simulink model "My_Model"  (R2022a)
settings: Solver=VariableStepAuto  StartTime=0.0  StopTime=10.0  RelTol=1e-3
libraries: neural x1294, spsSeriesRLCBranchLib x16, spsDiodeLib x14, spsMosfetLib x9, spsVoltageMeasurementLib x9, powerlib_extras x8, spsThreePhaseVIMeasurementLib x7, spsCurrentMeasurementLib x4, spsPVArrayLib x4, spsPWMGeneratorDCDCLib x4, spsTHDLib x4, spsThreePhaseParallelRLCBranchLib x3
(part 18 of 41)

== system My_Model/Subsystem1/Custom Neural Network1/Layer 5/IW{5,1} ==
  "pd{5,1}" : Inport  PortDimensions=2
      mask Display: e = 0.06;c1 = [120 230 180]/255;c2 = ([120 230 180]+0)/(256+128);c3 = ([120 230 180]+128)/(256+128);patch([0 1 1 0],[0 0 1 1],c1);patch([0 1 1 1-e 1-e 0+e],[0 0 1 1-e 0+e 0+e],c2);patch([0 0 1 1-e 0+e 0+e],[0 1 1 1-e 1-e 0+e],c3);plot([0 1 1 0 0],[0 0 1 1 0]);
  "IW{5,1}(1,:)'" : Constant  Value=[-0.01556453275093380543558918560620440985076129436492919921875;5.4972936922844959435792422386413136337068863213062286376953125e-05]
      mask Display: e = 0.06;c1 = [120 150 230]/255;c2 = ([120 150 230]+0)/383;c3 = ([120 150 230]+128)/383;patch([0 1 1 0],[0 0 1 1],c1);patch([0 1 1 1-e 1-e 0+e],[0 0 1 1-e 0+e 0+e],c2);patch([0 0 1 1-e 0+e 0+e],[0 1 1 1-e 1-e 0+e],c3);plot([0 1 1 0 0],[0 0 1 1 0]);disp('Weights');
  "IW{5,1}(2,:)'" : Constant  Value=[-0.00943826331659743111845983776220236904919147491455078125;-0.0251008390325845910651114678557860315777361392974853515625]
      mask Display: e = 0.06;c1 = [120 150 230]/255;c2 = ([120 150 230]+0)/383;c3 = ([120 150 230]+128)/383;patch([0 1 1 0],[0 0 1 1],c1);patch([0 1 1 1-e 1-e 0+e],[0 0 1 1-e 0+e 0+e],c2);patch([0 0 1 1-e 0+e 0+e],[0 1 1 1-e 1-e 0+e],c3);plot([0 1 1 0 0],[0 0 1 1 0]);disp('Weights');
  "IW{5,1}(3,:)'" : Constant  Value=[0.001691875226755712967319222883588736294768750667572021484375;0.01000054813071515023847890546448979876004159450531005859375]
      mask Display: e = 0.06;c1 = [120 150 230]/255;c2 = ([120 150 230]+0)/383;c3 = ([120 150 230]+128)/383;patch([0 1 1 0],[0 0 1 1],c1);patch([0 1 1 1-e 1-e 0+e],[0 0 1 1-e 0+e 0+e],c2);patch([0 0 1 1-e 0+e 0+e],[0 1 1 1-e 1-e 0+e],c3);plot([0 1 1 0 0],[0 0 1 1 0]);disp('Weights');
  "IW{5,1}(4,:)'" : Constant  Value=[0.00932793326903941753813764847791389911435544490814208984375;0.01364668381544361687451871745224707410670816898345947265625]
      mask Display: e = 0.06;c1 = [120 150 230]/255;c2 = ([120 150 230]+0)/383;c3 = ([120 150 230]+128)/383;patch([0 1 1 0],[0 0 1 1],c1);patch([0 1 1 1-e 1-e 0+e],[0 0 1 1-e 0+e 0+e],c2);patch([0 0 1 1-e 0+e 0+e],[0 1 1 1-e 1-e 0+e],c3);plot([0 1 1 0 0],[0 0 1 1 0]);disp('Weights');
  "IW{5,1}(5,:)'" : Constant  Value=[-0.002392923396249546121039575297118062735535204410552978515625;-0.026184378671104908964384350156251457519829273223876953125]
      mask Display: e = 0.06;c1 = [120 150 230]/255;c2 = ([120 150 230]+0)/383;c3 = ([120 150 230]+128)/383;patch([0 1 1 0],[0 0 1 1],c1);patch([0 1 1 1-e 1-e 0+e],[0 0 1 1-e 0+e 0+e],c2);patch([0 0 1 1-e 0+e 0+e],[0 1 1 1-e 1-e 0+e],c3);plot([0 1 1 0 0],[0 0 1 1 0]);disp('Weights');
  Mux : Mux  Inputs=5
      mask Display: e = 0.06;c1 = [120 150 230]/255;c2 = ([120 150 230]+0)/383;c3 = ([120 150 230]+128)/383;patch([0 1 1 0],[0 0 1 1],c1);patch([0 1 1 1-e 1-e 0+e],[0 0 1 1-e 0+e 0+e],c2);patch([0 0 1 1-e 0+e 0+e],[0 1 1 1-e 1-e 0+e],c3);plot([0 1 1 0 0],[0 0 1 1 0]);disp('Mux');
  dotprod{1..5} (5 alike) : neural/Weight Functions/dotprod
  "iz{5,1}" : Outport
      mask Display: e = 0.06;c1 = [120 230 180]/255;c2 = ([120 230 180]+0)/(256+128);c3 = ([120 230 180]+128)/(256+128);patch([0 1 1 0],[0 0 1 1],c1);patch([0 1 1 1-e 1-e 0+e],[0 0 1 1-e 0+e 0+e],c2);patch([0 0 1 1-e 0+e 0+e],[0 1 1 1-e 1-e 0+e],c3);plot([0 1 1 0 0],[0 0 1 1 0]);
  wires:
  Mux/1 -> "iz{5,1}"/1
  dotprod5/1 -> Mux/5
  "IW{5,1}(5,:)'"/1 -> dotprod5/1
  dotprod4/1 -> Mux/4
  "IW{5,1}(4,:)'"/1 -> dotprod4/1
  dotprod3/1 -> Mux/3
  "IW{5,1}(3,:)'"/1 -> dotprod3/1
  dotprod2/1 -> Mux/2
  "IW{5,1}(2,:)'"/1 -> dotprod2/1
  dotprod1/1 -> Mux/1
  "pd{5,1}"/1 -> dotprod5/2, dotprod4/2, dotprod3/2, dotprod2/2, dotprod1/2
  "IW{5,1}(1,:)'"/1 -> dotprod1/1

== system My_Model/Subsystem1/Custom Neural Network1/Layer 5/LW{5,1} ==
  "ad{5,1}" : Inport  PortDimensions=5
      mask Display: e = 0.06;c1 = [120 230 180]/255;c2 = ([120 230 180]+0)/(256+128);c3 = ([120 230 180]+128)/(256+128);patch([0 1 1 0],[0 0 1 1],c1);patch([0 1 1 1-e 1-e 0+e],[0 0 1 1-e 0+e 0+e],c2);patch([0 0 1 1-e 0+e 0+e],[0 1 1 1-e 1-e 0+e],c3);plot([0 1 1 0 0],[0 0 1 1 0]);
  "IW{5,1}(1,:)'" : Constant  Value=[0.198320715847589756908320168804493732750415802001953125;-0.76675737162833801363603924983181059360504150390625;1.08955055179509141538574112928472459316253662109375;-0.2713503308288773840928342906408943235874176025390625;-0.6565776104818485947589579154737293720245361328125]
      mask Display: e = 0.06;c1 = [120 150 230]/255;c2 = ([120 150 230]+0)/383;c3 = ([120 150 230]+128)/383;patch([0 1 1 0],[0 0 1 1],c1);patch([0 1 1 1-e 1-e 0+e],[0 0 1 1-e 0+e 0+e],c2);patch([0 0 1 1-e 0+e 0+e],[0 1 1 1-e 1-e 0+e],c3);plot([0 1 1 0 0],[0 0 1 1 0]);disp('weights');
  "IW{5,1}(2,:)'" : Constant  Value=[0.0779959574242100328600457714856020174920558929443359375;-0.10003962086747404669484495798315037973225116729736328125;1.0731906798303751937595507115474902093410491943359375;0.000534257552850309481821955426283921042340807616710662841796875;0.413508652564843204313405067296116612851619720458984375]
      mask Display: e = 0.06;c1 = [120 150 230]/255;c2 = ([120 150 230]+0)/383;c3 = ([120 150 230]+128)/383;patch([0 1 1 0],[0 0 1 1],c1);patch([0 1 1 1-e 1-e 0+e],[0 0 1 1-e 0+e 0+e],c2);patch([0 0 1 1-e 0+e 0+e],[0 1 1 1-e 1-e 0+e],c3);plot([0 1 1 0 0],[0 0 1 1 0]);disp('weights');
  "IW{5,1}(3,:)'" : Constant  Value=[0.0464276696923932308269655777621665038168430328369140625;-0.191886394147698258194623122108168900012969970703125;-0.3521992231427344410832347421091981232166290283203125;0.64609742274914416793052396315033547580242156982421875;1.0262809271427844048929500786471180617809295654296875]
      mask Display: e = 0.06;c1 = [120 150 230]/255;c2 = ([120 150 230]+0)/383;c3 = ([120 150 230]+128)/383;patch([0 1 1 0],[0 0 1 1],c1);patch([0 1 1 1-e 1-e 0+e],[0 0 1 1-e 0+e 0+e],c2);patch([0 0 1 1-e 0+e 0+e],[0 1 1 1-e 1-e 0+e],c3);plot([0 1 1 0 0],[0 0 1 1 0]);disp('weights');
  "IW{5,1}(4,:)'" : Constant  Value=[0.98375907186508115831458098909934051334857940673828125;-0.1830940829093224142543050447784480638802051544189453125;0.9452581550422547440604148505371995270252227783203125;-0.320309813947215082929886875717784278094768524169921875;-0.73154898069945961669446887754020281136035919189453125]
      mask Display: e = 0.06;c1 = [120 150 230]/255;c2 = ([120 150 230]+0)/383;c3 = ([120 150 230]+128)/383;patch([0 1 1 0],[0 0 1 1],c1);patch([0 1 1 1-e 1-e 0+e],[0 0 1 1-e 0+e 0+e],c2);patch([0 0 1 1-e 0+e 0+e],[0 1 1 1-e 1-e 0+e],c3);plot([0 1 1 0 0],[0 0 1 1 0]);disp('weights');
  "IW{5,1}(5,:)'" : Constant  Value=[0.25564330598621010093296490595093928277492523193359375;-0.09094017318610138345125193382045836187899112701416015625;-0.436280716359431774975519147119484841823577880859375;-0.348300498410330672260926121452939696609973907470703125;0.93083543676170144021142505152965895831584930419921875]
      mask Display: e = 0.06;c1 = [120 150 230]/255;c2 = ([120 150 230]+0)/383;c3 = ([120 150 230]+128)/383;patch([0 1 1 0],[0 0 1 1],c1);patch([0 1 1 1-e 1-e 0+e],[0 0 1 1-e 0+e 0+e],c2);patch([0 0 1 1-e 0+e 0+e],[0 1 1 1-e 1-e 0+e],c3);plot([0 1 1 0 0],[0 0 1 1 0]);disp('weights');
  Mux : Mux  Inputs=5
      mask Display: e = 0.06;c1 = [120 150 230]/255;c2 = ([120 150 230]+0)/383;c3 = ([120 150 230]+128)/383;patch([0 1 1 0],[0 0 1 1],c1);patch([0 1 1 1-e 1-e 0+e],[0 0 1 1-e 0+e 0+e],c2);patch([0 0 1 1-e 0+e 0+e],[0 1 1 1-e 1-e 0+e],c3);plot([0 1 1 0 0],[0 0 1 1 0]);disp('Mux');
  dotprod{1..5} (5 alike) : neural/Weight Functions/dotprod
  "lz{5,1}" : Outport
      mask Display: e = 0.06;c1 = [120 230 180]/255;c2 = ([120 230 180]+0)/(256+128);c3 = ([120 230 180]+128)/(256+128);patch([0 1 1 0],[0 0 1 1],c1);patch([0 1 1 1-e 1-e 0+e],[0 0 1 1-e 0+e 0+e],c2);patch([0 0 1 1-e 0+e 0+e],[0 1 1 1-e 1-e 0+e],c3);plot([0 1 1 0 0],[0 0 1 1 0]);
  wires:
  Mux/1 -> "lz{5,1}"/1
  dotprod5/1 -> Mux/5
  "IW{5,1}(5,:)'"/1 -> dotprod5/1
  dotprod4/1 -> Mux/4
  "IW{5,1}(4,:)'"/1 -> dotprod4/1
  dotprod3/1 -> Mux/3
  "IW{5,1}(3,:)'"/1 -> dotprod3/1
  dotprod2/1 -> Mux/2
  "IW{5,1}(2,:)'"/1 -> dotprod2/1
  dotprod1/1 -> Mux/1
  "ad{5,1}"/1 -> dotprod5/2, dotprod4/2, dotprod3/2, dotprod2/2, dotprod1/2
  "IW{5,1}(1,:)'"/1 -> dotprod1/1

== system My_Model/Subsystem1/Custom Neural Network1/Layer 5/LW{5,2} ==
  "ad{5,2}" : Inport  PortDimensions=20
      mask Display: e = 0.06;c1 = [120 230 180]/255;c2 = ([120 230 180]+0)/(256+128);c3 = ([120 230 180]+128)/(256+128);patch([0 1 1 0],[0 0 1 1],c1);patch([0 1 1 1-e 1-e 0+e],[0 0 1 1-e 0+e 0+e],c2);patch([0 0 1 1-e 0+e 0+e],[0 1 1 1-e 1-e 0+e],c3);plot([0 1 1 0 0],[0 0 1 1 0]);
  "IW{5,2}(1,:)'" : Constant  Value=[-0.1684832167230098931565152042821864597499370574951171875;-0.158311694875728659059888059346121735870838165283203125;0.03144274628571579188740514609889942221343517303466796875;0.58926160433097063418017569347284734249114990234375;0.9422248117175568982162303655059076845645904541015625;-0.7561502004801388121535410391516052186489105224609375;0.2469253151334374896119783215908682905137538909912109375;0.36342459520089909208451217637048102915287017822265625;0.34969813386813874966918547215755097568035125732421875;-0.75124035402883071466106912339455448091030120849609375;-1.200718051335563085757485168869607150554656982421875;1.0762949692530996426143019562005065381526947021484375;1.1023353041015584441453256658860482275485992431640625;-0.267493816107898629841344018132076598703861236572265625;-0.81521522741978114101613073216867633163928985595703125;-1.037383369655141773790774095687083899974822998046875;0.27978157127544756033188377841725014150142669677734375;1.1838317043498267633339082749444060027599334716796875;-0.2358763441495083379439989812453859485685825347900390625;0.1897216833489547838098587817512452602386474609375]
      mask Display: e = 0.06;c1 = [120 150 230]/255;c2 = ([120 150 230]+0)/383;c3 = ([120 150 230]+128)/383;patch([0 1 1 0],[0 0 1 1],c1);patch([0 1 1 1-e 1-e 0+e],[0 0 1 1-e 0+e 0+e],c2);patch([0 0 1 1-e 0+e 0+e],[0 1 1 1-e 1-e 0+e],c3);plot([0 1 1 0 0],[0 0 1 1 0]);disp('weights');
  "IW{5,2}(2,:)'" : Constant  Value=[0.5812767377017793446469795526354573667049407958984375;-0.58065264983084985406236455673933960497379302978515625;-0.53889712674579726137125135210226289927959442138671875;0.455212321068005021373892304836772382259368896484375;0.381546915238895001376562277073389850556850433349609375;-0.9898117600722893261178114698850549757480621337890625;-0.036772065646242212133554261299650534056127071380615234375;0.344368316606951607727893360788584686815738677978515625;0.37959793987010959082084582405514083802700042724609375;0.99126589260002884174127757432870566844940185546875;-0.99833075074241206525726965992362238466739654541015625;0.934549989284991777793720757472328841686248779296875;-0.042023664020545518915650262670169468037784099578857421875;-0.50812566427233230026416777036502026021480560302734375;0.8581247546815966575906031721387989819049835205078125;-1.1160299752370683723512456708704121410846710205078125;-0.26941229108102737743735133335576392710208892822265625;-0.45029337265439028925584352691657841205596923828125;-0.12270439641062207136723571920811082236468791961669921875;0.492220096251096694839333167692529968917369842529296875]
      mask Display: e = 0.06;c1 = [120 150 230]/255;c2 = ([120 150 230]+0)/383;c3 = ([120 150 230]+128)/383;patch([0 1 1 0],[0 0 1 1],c1);patch([0 1 1 1-e 1-e 0+e],[0 0 1 1-e 0+e 0+e],c2);patch([0 0 1 1-e 0+e 0+e],[0 1 1 1-e 1-e 0+e],c3);plot([0 1 1 0 0],[0 0 1 1 0]);disp('weights');
  "IW{5,2}(3,:)'" : Constant  Value=[-0.1648517007952392809944086593532119877636432647705078125;-0.35915922041747305737402484737685881555080413818359375;-1.1402981796676645576127384629216976463794708251953125;-0.27685202188738078366014860876020975410938262939453125;0.392134378238151837248182118855766020715236663818359375;1.217305601499260259146240059635601937770843505859375;0.4563227505947524687002214704989455640316009521484375;-0.60795376192282446492498593215714208781719207763671875;-1.2351866808087625937417897148407064378261566162109375;-0.304290353056002105258670553666888736188411712646484375;-0.0281049809085356337712280350160654052160680294036865234375;-0.07228816906939468378556767902409774251282215118408203125;-0.0274877397507839980883570518699343665502965450286865234375;0.2313225831755712780246625470681465230882167816162109375;-0.44365232337631421710710810657474212348461151123046875;-0.5191098010197474632576586373033933341503143310546875;0.310823132335534768611040590258198790252208709716796875;0.7164023227649478631207102807820774614810943603515625;0.6809741715773840464720478848903439939022064208984375;-0.8507340797159843592822880964376963675022125244140625]
      mask Display: e = 0.06;c1 = [120 150 230]/255;c2 = ([120 150 230]+0)/383;c3 = ([120 150 230]+128)/383;patch([0 1 1 0],[0 0 1 1],c1);patch([0 1 1 1-e 1-e 0+e],[0 0 1 1-e 0+e 0+e],c2);patch([0 0 1 1-e 0+e 0+e],[0 1 1 1-e 1-e 0+e],c3);plot([0 1 1 0 0],[0 0 1 1 0]);disp('weights');
  "IW{5,2}(4,:)'" : Constant  Value=[0.6350658920207326030293870644527487456798553466796875;0.78502750463090731347648443261277861893177032470703125;0.762793473272745270463701672269962728023529052734375;0.37784362235353541326077220219303853809833526611328125;-0.192588124811389704849062809444149024784564971923828125;0.77541139946467751986602934266556985676288604736328125;0.61832300773275472582923839581781066954135894775390625;-0.7310412564267725343825077288784086704254150390625;-0.5449629474225596847958286161883734166622161865234375;1.1444776365309892174337846881826408207416534423828125;-0.050150885878106822579614032520112232305109500885009765625;0.6877296369174070722607439165585674345493316650390625;-0.39848068932220515048214792841463349759578704833984375;0.236964859673772565429317182861268520355224609375;0.1226832073435409620199010305441333912312984466552734375;-0.76214660363326203196265851147472858428955078125;-0.98776348259720714306553190908743999898433685302734375;1.055032779571795753525975669617764651775360107421875;-1.09102444565933875963992250035516917705535888671875;0.79757981845308645318937124102376401424407958984375]
      mask Display: e = 0.06;c1 = [120 150 230]/255;c2 = ([120 150 230]+0)/383;c3 = ([120 150 230]+128)/383;patch([0 1 1 0],[0 0 1 1],c1);patch([0 1 1 1-e 1-e 0+e],[0 0 1 1-e 0+e 0+e],c2);patch([0 0 1 1-e 0+e 0+e],[0 1 1 1-e 1-e 0+e],c3);plot([0 1 1 0 0],[0 0 1 1 0]);disp('weights');
  "IW{5,2}(5,:)'" : Constant  Value=[-0.529727220867986403618488111533224582672119140625;0.70651597831416446116037377578322775661945343017578125;-1.047591944087713500266545452177524566650390625;-0.405419647769215740762405175701132975518703460693359375;-1.0223374069193038593539313296787440776824951171875;-0.66965658547109130349639372070669196546077728271484375;-0.291852462499349540880899667172343470156192779541015625;0.65359162375761403751539546647109091281890869140625;-0.16324908144528327280653456909931264817714691162109375;-0.6050588281762083742165714284055866301059722900390625;-0.1199441337484412339886574727643164806067943572998046875;-0.532459193107392980692793571506626904010772705078125;0.5539672672926834184892186385695822536945343017578125;-0.65825035682826638083753323371638543903827667236328125;-0.469079745718143925614640465937554836273193359375;-0.961416751874887065554275977774523198604583740234375;-1.0711718673191363837560174943064339458942413330078125;0.65147983239813544997787175816483795642852783203125;-0.033235468255095899914319801382589503191411495208740234375;-0.69039012441932900987495713707176037132740020751953125]
      mask Display: e = 0.06;c1 = [120 150 230]/255;c2 = ([120 150 230]+0)/383;c3 = ([120 150 230]+128)/383;patch([0 1 1 0],[0 0 1 1],c1);patch([0 1 1 1-e 1-e 0+e],[0 0 1 1-e 0+e 0+e],c2);patch([0 0 1 1-e 0+e 0+e],[0 1 1 1-e 1-e 0+e],c3);plot([0 1 1 0 0],[0 0 1 1 0]);disp('weights');
  Mux : Mux  Inputs=5
      mask Display: e = 0.06;c1 = [120 150 230]/255;c2 = ([120 150 230]+0)/383;c3 = ([120 150 230]+128)/383;patch([0 1 1 0],[0 0 1 1],c1);patch([0 1 1 1-e 1-e 0+e],[0 0 1 1-e 0+e 0+e],c2);patch([0 0 1 1-e 0+e 0+e],[0 1 1 1-e 1-e 0+e],c3);plot([0 1 1 0 0],[0 0 1 1 0]);disp('Mux');
  dotprod{1..5} (5 alike) : neural/Weight Functions/dotprod
  "lz{5,2}" : Outport
      mask Display: e = 0.06;c1 = [120 230 180]/255;c2 = ([120 230 180]+0)/(256+128);c3 = ([120 230 180]+128)/(256+128);patch([0 1 1 0],[0 0 1 1],c1);patch([0 1 1 1-e 1-e 0+e],[0 0 1 1-e 0+e 0+e],c2);patch([0 0 1 1-e 0+e 0+e],[0 1 1 1-e 1-e 0+e],c3);plot([0 1 1 0 0],[0 0 1 1 0]);
  wires:
  Mux/1 -> "lz{5,2}"/1
  dotprod5/1 -> Mux/5
  "IW{5,2}(5,:)'"/1 -> dotprod5/1
  dotprod4/1 -> Mux/4
  "IW{5,2}(4,:)'"/1 -> dotprod4/1
  dotprod3/1 -> Mux/3
  "IW{5,2}(3,:)'"/1 -> dotprod3/1
  dotprod2/1 -> Mux/2
  "IW{5,2}(2,:)'"/1 -> dotprod2/1
  dotprod1/1 -> Mux/1
  "ad{5,2}"/1 -> dotprod5/2, dotprod4/2, dotprod3/2, dotprod2/2, dotprod1/2
  "IW{5,2}(1,:)'"/1 -> dotprod1/1

== system My_Model/Subsystem1/Custom Neural Network1/Layer 5/LW{5,3} ==
  "ad{5,3}" : Inport  PortDimensions=30
      mask Display: e = 0.06;c1 = [120 230 180]/255;c2 = ([120 230 180]+0)/(256+128);c3 = ([120 230 180]+128)/(256+128);patch([0 1 1 0],[0 0 1 1],c1);patch([0 1 1 1-e 1-e 0+e],[0 0 1 1-e 0+e 0+e],c2);patch([0 0 1 1-e 0+e 0+e],[0 1 1 1-e 1-e 0+e],c3);plot([0 1 1 0 0],[0 0 1 1 0]);
  "IW{5,3}(1,:)'" : Constant  Value=[0.06976811311634777135193274943958385847508907318115234375;-0.8904230643978845449737491435371339321136474609375;-0.1775310035236150330018034537715720944106578826904296875;1.0090421076723676829800524501479230821132659912109375;-0.417702847790847264786151527005131356418132781982421875;0.7097914782253080812068901650491170585155487060546875;0.63612699655700932765967081650160253047943115234375;0.288855656116090597773649051305255852639675140380859375;0.95976629130618007490483023502747528254985809326171875;-0.7905788500602326518418294654111377894878387451171875;0.990929063210639782255384488962590694427490234375;0.469011925257395489996525839160312898457050323486328125;-0.7636022398618582673890387013670988380908966064453125;-0.5749085722730615799491715733893215656280517578125;-0.05474432168254728114931140225962735712528228759765625;-0.25277578610224626931568536747363395988941192626953125;-0.28171406869540194239931452102609910070896148681640625;-0.474471903162546893018003402175963856279850006103515625;1.0713990955559704598698544941726140677928924560546875;-0.74396982003213396605900697977631352841854095458984375;-1.0225688834784014691337006297544576227664947509765625;-1.176604496566949098479426538688130676746368408203125;0.31006559905746378102975313595379702746868133544921875;0.022347790486875462878657572218799032270908355712890625;-0.5299835679185707082439193982281722128391265869140625;0.30973067574931734124987769973813556134700775146484375;0.476067198470006613941762907415977679193019866943359375;-0.85039389662740838549126465295557864010334014892578125;-0.88214826493247688876664369672653265297412872314453125;0.204961332422772202210836667291005142033100128173828125]
      mask Display: e = 0.06;c1 = [120 150 230]/255;c2 = ([120 150 230]+0)/383;c3 = ([120 150 230]+128)/383;patch([0 1 1 0],[0 0 1 1],c1);patch([0 1 1 1-e 1-e 0+e],[0 0 1 1-e 0+e 0+e],c2);patch([0 0 1 1-e 0+e 0+e],[0 1 1 1-e 1-e 0+e],c3);plot([0 1 1 0 0],[0 0 1 1 0]);disp('weights');
  "IW{5,3}(2,:)'" : Constant  Value=[1.02607673757031658823279940406791865825653076171875;-0.67061548482769761658772722512367181479930877685546875;-0.79841600024922321221509946553851477801799774169921875;-1.0723128333001190615192399491206742823123931884765625;1.06628933443160622829282146994955837726593017578125;-0.0179940190794609967961381613577032112516462802886962890625;-0.305889185839444965875344450978445820510387420654296875;0.333052790045151481113094860120327211916446685791015625;0.51567508404394157839334411619347520172595977783203125;1.0714210085002064953840772432158701121807098388671875;0.004025141173272854706877144082000086200423538684844970703125;-1.0474116032867477610324158376897685229778289794921875;0.18241219288394960873489480945863761007785797119140625;0.473496610911463611248706229162053205072879791259765625;-0.72500253650374890668217631173320114612579345703125;0.80219779574011995659787999102263711392879486083984375;-0.046275533330277764110238791772644617594778537750244140625;0.334934409051642401067283572047017514705657958984375;-0.01243645460155369357468924107479324447922408580780029296875;-0.364996573067974339199537325839628465473651885986328125;-0.492963770259384592709039907276746816933155059814453125;-0.66010196944313437317219950273283757269382476806640625;-0.32028917197858552956546418499783612787723541259765625;-0.71569019611373552169908407449838705360889434814453125;0.10286137044281462582517860937514342367649078369140625;-1.0968709513793584164886851795017719268798828125;1.1294113476131968365478996929596178233623504638671875;0.2232226246753103160447295749690965749323368072509765625;0.87301676376418624325737027902505360543727874755859375;0.5910374993698550571963323818636126816272735595703125]
      mask Display: e = 0.06;c1 = [120 150 230]/255;c2 = ([120 150 230]+0)/383;c3 = ([120 150 230]+128)/383;patch([0 1 1 0],[0 0 1 1],c1);patch([0 1 1 1-e 1-e 0+e],[0 0 1 1-e 0+e 0+e],c2);patch([0 0 1 1-e 0+e 0+e],[0 1 1 1-e 1-e 0+e],c3);plot([0 1 1 0 0],[0 0 1 1 0]);disp('weights');
  "IW{5,3}(3,:)'" : Constant  Value=[0.911956403472287124856165974051691591739654541015625;0.73120964429517532057190010164049454033374786376953125;-0.19239066195573795159390328990411944687366485595703125;0.1445667439966855372102116916721570305526256561279296875;-0.0033231170370225369438410556455210098647512495517730712890625;-0.59830843381236054057126239058561623096466064453125;0.408667666911742111235383845269097946584224700927734375;-0.831982576988268274220672537921927869319915771484375;0.3517587454973412075531769005465321242809295654296875;-0.35896977430946808151901450401055626571178436279296875;-0.3235074744318164885470423541846685111522674560546875;-0.0239287379100967985412484750895600882358849048614501953125;0.281367055026232437686672938070842064917087554931640625;-0.3788843582453995662007173450547270476818084716796875;0.0342707683378646044136672799140796996653079986572265625;0.5856034280158539662153316385229118168354034423828125;-0.8748270322766675821668513890472240746021270751953125;-0.58722513700674217052011272244271822273731231689453125;0.51864705919583597992783552399487234652042388916015625;0.144311428807947061958572021467261947691440582275390625;-0.1661982997721902222121315162439714185893535614013671875;0.652477698383433502016259808442555367946624755859375;-0.408825238471636709380874208363820798695087432861328125;1.206433139098817886036840718588791787624359130859375;-1.1799999057322494433464044050197117030620574951171875;-0.82861375039548634813257876885472796857357025146484375;0.81000415733947195295883147991844452917575836181640625;1.047012487125788648967272820300422608852386474609375;-1.023882188725524056138738160370849072933197021484375;-1.0018472902214641262474970062612555921077728271484375]
      mask Display: e = 0.06;c1 = [120 150 230]/255;c2 = ([120 150 230]+0)/383;c3 = ([120 150 230]+128)/383;patch([0 1 1 0],[0 0 1 1],c1);patch([0 1 1 1-e 1-e 0+e],[0 0 1 1-e 0+e 0+e],c2);patch([0 0 1 1-e 0+e 0+e],[0 1 1 1-e 1-e 0+e],c3);plot([0 1 1 0 0],[0 0 1 1 0]);disp('weights');
  "IW{5,3}(4,:)'" : Constant  Value=[0.131501480971123518859400292058126069605350494384765625;0.66279150960733546060765775109757669270038604736328125;0.63884422027081166906015141648822464048862457275390625;0.72909653390863382593778396767447702586650848388671875;-0.90546465435929246456936425602179951965808868408203125;0.391882833098547156414070968821761198341846466064453125;0.1911551389353061403131306406066869385540485382080078125;0.487794714092320003118175009149126708507537841796875;-1.070986344739118134583577557350508868694305419921875;-0.01148351199106119845116946720509076840244233608245849609375;0.09598816393457938744848689793798257596790790557861328125;-0.80822404326281083175587127698236145079135894775390625;0.79272828448982390892041394181433133780956268310546875;0.581678827825609090496072894893586635589599609375;0.5553662964094172593831899575889110565185546875;0.8806441595504901354019011705531738698482513427734375;0.304304805080709395159743735348456539213657379150390625;-0.399632884153812373284608838730491697788238525390625;0.47036869694372895889245000944356434047222137451171875;-0.370420330664536001652464847211376763880252838134765625;1.0757632659218800963429885086952708661556243896484375;0.499792790216292026617139754307572729885578155517578125;-1.1249752973375908293718339336919598281383514404296875;-0.99957650870437009249513948816456831991672515869140625;-0.495562736705339734744057977877673693001270294189453125;0.223154680657428994283719703162205405533313751220703125;0.84780150873613013828844486852176487445831298828125;-0.77027674138608392961913295948761515319347381591796875;0.58493918341868489374490991394850425422191619873046875;0.76452357438165041703115321070072241127490997314453125]
      mask Display: e = 0.06;c1 = [120 150 230]/255;c2 = ([120 150 230]+0)/383;c3 = ([120 150 230]+128)/383;patch([0 1 1 0],[0 0 1 1],c1);patch([0 1 1 1-e 1-e 0+e],[0 0 1 1-e 0+e 0+e],c2);patch([0 0 1 1-e 0+e 0+e],[0 1 1 1-e 1-e 0+e],c3);plot([0 1 1 0 0],[0 0 1 1 0]);disp('weights');
  "IW{5,3}(5,:)'" : Constant  Value=[-0.7949475215612575862422772843274287879467010498046875;-0.78705521859511595739178346775588579475879669189453125;-0.14105485824722363563665794572443701326847076416015625;-0.98435689700852524453011938021518290042877197265625;-0.9279846614916344993417851583217270672321319580078125;0.1497052841760106167701138701886520721018314361572265625;1.014994471582784552055045423912815749645233154296875;0.33012334302225154747389979092986322939395904541015625;0.058575433865315724990541212946482119150459766387939453125;-0.9220886386425470870875642503960989415645599365234375;-0.1755625087052014310362579863067367114126682281494140625;0.724758853697351046463381862849928438663482666015625;-0.35773147511886149718662863961071707308292388916015625;0.57157465399289175689290232185157947242259979248046875;0.487261121070496849849718046243651770055294036865234375;-0.91283372493046233131508415681309998035430908203125;-0.0327107793084950027040491704610758461058139801025390625;0.46507670819269986139943284797482192516326904296875;-0.50221145378164033790113762734108604490756988525390625;0.449225827706557445662127747709746472537517547607421875;1.0459019683752279750166280791745521128177642822265625;-0.5375601512357921496487733747926540672779083251953125;0.2243261330991283275526626539431163109838962554931640625;0.3222282816435677599287146222195588052272796630859375;0.6834030649040780946990025768172927200794219970703125;-1.07651202231523424046599757275544106960296630859375;-0.1531612267181061415310949769263970665633678436279296875;0.426535554950608908342246650136075913906097412109375;-0.7775472530073148647034031455405056476593017578125;-0.01644391036485957913182431866516708396375179290771484375]
      mask Display: e = 0.06;c1 = [120 150 230]/255;c2 = ([120 150 230]+0)/383;c3 = ([120 150 230]+128)/383;patch([0 1 1 0],[0 0 1 1],c1);patch([0 1 1 1-e 1-e 0+e],[0 0 1 1-e 0+e 0+e],c2);patch([0 0 1 1-e 0+e 0+e],[0 1 1 1-e 1-e 0+e],c3);plot([0 1 1 0 0],[0 0 1 1 0]);disp('weights');
  Mux : Mux  Inputs=5
      mask Display: e = 0.06;c1 = [120 150 230]/255;c2 = ([120 150 230]+0)/383;c3 = ([120 150 230]+128)/383;patch([0 1 1 0],[0 0 1 1],c1);patch([0 1 1 1-e 1-e 0+e],[0 0 1 1-e 0+e 0+e],c2);patch([0 0 1 1-e 0+e 0+e],[0 1 1 1-e 1-e 0+e],c3);plot([0 1 1 0 0],[0 0 1 1 0]);disp('Mux');
  dotprod{1..5} (5 alike) : neural/Weight Functions/dotprod
  "lz{5,3}" : Outport
      mask Display: e = 0.06;c1 = [120 230 180]/255;c2 = ([120 230 180]+0)/(256+128);c3 = ([120 230 180]+128)/(256+128);patch([0 1 1 0],[0 0 1 1],c1);patch([0 1 1 1-e 1-e 0+e],[0 0 1 1-e 0+e 0+e],c2);patch([0 0 1 1-e 0+e 0+e],[0 1 1 1-e 1-e 0+e],c3);plot([0 1 1 0 0],[0 0 1 1 0]);
  wires:
  Mux/1 -> "lz{5,3}"/1
  dotprod5/1 -> Mux/5
  "IW{5,3}(5,:)'"/1 -> dotprod5/1
  dotprod4/1 -> Mux/4
  "IW{5,3}(4,:)'"/1 -> dotprod4/1
  dotprod3/1 -> Mux/3
  "IW{5,3}(3,:)'"/1 -> dotprod3/1
  dotprod2/1 -> Mux/2
  "IW{5,3}(2,:)'"/1 -> dotprod2/1
  dotprod1/1 -> Mux/1
  "ad{5,3}"/1 -> dotprod5/2, dotprod4/2, dotprod3/2, dotprod2/2, dotprod1/2
  "IW{5,3}(1,:)'"/1 -> dotprod1/1

== system My_Model/Subsystem1/Custom Neural Network1/Layer 5/LW{5,4} ==
  "ad{5,4}" : Inport  PortDimensions=20
      mask Display: e = 0.06;c1 = [120 230 180]/255;c2 = ([120 230 180]+0)/(256+128);c3 = ([120 230 180]+128)/(256+128);patch([0 1 1 0],[0 0 1 1],c1);patch([0 1 1 1-e 1-e 0+e],[0 0 1 1-e 0+e 0+e],c2);patch([0 0 1 1-e 0+e 0+e],[0 1 1 1-e 1-e 0+e],c3);plot([0 1 1 0 0],[0 0 1 1 0]);
  "IW{5,4}(1,:)'" : Constant  Value=[-0.1060894698163271920865469155614846386015415191650390625;1.0233811764657947396273129925248213112354278564453125;0.06417670731337622724854696798502118326723575592041015625;-0.59476674886658431606889507747837342321872711181640625;-1.085331649006446408378678825101815164089202880859375;0.5139773218494132489553294362849555909633636474609375;-0.1712255413970973083603865916302311234176158905029296875;-0.68605955505504156999307951991795562207698822021484375;0.41369772297360885016104248279589228332042694091796875;-0.7240871836100006841974163762643001973628997802734375;0.76421097622566680485078904894180595874786376953125;-0.7427364711749520065353635800420306622982025146484375;0.86474621536416618194920147288939915597438812255859375;-0.3648710491278046585961192249669693410396575927734375;0.29797295284211167132326636419747956097126007080078125;0.336000844551395172477015194090199656784534454345703125;-0.096908414214406379816324488274403847754001617431640625;0.5464771883025638654629574375576339662075042724609375;0.038151340577739001336254887064569629728794097900390625;0.09259862232598194131671931472737924195826053619384765625]
      mask Display: e = 0.06;c1 = [120 150 230]/255;c2 = ([120 150 230]+0)/383;c3 = ([120 150 230]+128)/383;patch([0 1 1 0],[0 0 1 1],c1);patch([0 1 1 1-e 1-e 0+e],[0 0 1 1-e 0+e 0+e],c2);patch([0 0 1 1-e 0+e 0+e],[0 1 1 1-e 1-e 0+e],c3);plot([0 1 1 0 0],[0 0 1 1 0]);disp('weights');
  "IW{5,4}(2,:)'" : Constant  Value=[-0.73449912405823936101256776964874006807804107666015625;-0.171822983720469668611485758447088301181793212890625;-0.60308195203195769096282674581743776798248291015625;0.9529020217517791824235473541193641722202301025390625;-0.79144474935493736023062183448928408324718475341796875;-0.371583516691538495724245194651302881538867950439453125;0.333234281418886280068392125031095929443836212158203125;0.62905521230362182460993381027947179973125457763671875;-0.9257327409476676649546789121814072132110595703125;0.59711214293720404899801224019029177725315093994140625;0.6220107656780415883446266889222897589206695556640625;1.1198087688821491969548560518887825310230255126953125;0.431944676138234784357194939730106852948665618896484375;-0.304375323158541488677286679376265965402126312255859375;-0.2823235379615940399133933169650845229625701904296875;-0.8672908144157762677650680416263639926910400390625;-0.5258466032150919122756249635131098330020904541015625;-0.39820909864451581317013051375397481024265289306640625;0.59827705992757584940733295297832228243350982666015625;0.755701895759301578436861746013164520263671875]
      mask Display: e = 0.06;c1 = [120 150 230]/255;c2 = ([120 150 230]+0)/383;c3 = ([120 150 230]+128)/383;patch([0 1 1 0],[0 0 1 1],c1);patch([0 1 1 1-e 1-e 0+e],[0 0 1 1-e 0+e 0+e],c2);patch([0 0 1 1-e 0+e 0+e],[0 1 1 1-e 1-e 0+e],c3);plot([0 1 1 0 0],[0 0 1 1 0]);disp('weights');
  "IW{5,4}(3,:)'" : Constant  Value=[-0.432095273224060216765707309605204500257968902587890625;-1.00529971143475460593208481441251933574676513671875;1.1481097277647573928760493799927644431591033935546875;0.91038684339439013282202495247474871575832366943359375;0.058244492840952129253384583762453985400497913360595703125;0.469012127005547452274214492717874236404895782470703125;-0.09236306596329087181818096041752141900360584259033203125;0.92986508373380949432629449802334420382976531982421875;-0.411140063932206534236257766679045744240283966064453125;-0.780493828111672893754757751594297587871551513671875;0.27589054546307145709960195745225064456462860107421875;0.84507444463074310458949867097544483840465545654296875;0.14807162439555898725274118987726978957653045654296875;-1.2544077282066494749557250543148256838321685791015625;1.0459215310743343874122501802048645913600921630859375;0.8273329588285907032485511081176809966564178466796875;-0.230533224480857779070674951071850955486297607421875;-0.64511002106111536846810849965550005435943603515625;0.040873751403180551278193632924740086309611797332763671875;0.233432165689983539547114332890487276017665863037109375]
      mask Display: e = 0.06;c1 = [120 150 230]/255;c2 = ([120 150 230]+0)/383;c3 = ([120 150 230]+128)/383;patch([0 1 1 0],[0 0 1 1],c1);patch([0 1 1 1-e 1-e 0+e],[0 0 1 1-e 0+e 0+e],c2);patch([0 0 1 1-e 0+e 0+e],[0 1 1 1-e 1-e 0+e],c3);plot([0 1 1 0 0],[0 0 1 1 0]);disp('weights');
  "IW{5,4}(4,:)'" : Constant  Value=[-0.10355905667129407243809424699065857566893100738525390625;0.3479126638571461427318354253657162189483642578125;-0.41149440776604817582295936517766676843166351318359375;-1.1169179085585458910401257526245899498462677001953125;0.2264442088889926096850757630818407051265239715576171875;-0.113788317635191316146148210464161820709705352783203125;0.00500235840824870582610461866579498746432363986968994140625;0.09745765714042686767015766235999763011932373046875;-0.615162276350938785896005356335081160068511962890625;0.499754962002299130130467119670356623828411102294921875;0.333631884822824076319847108607064001262187957763671875;0.9336478498228986122597916619270108640193939208984375;-0.982171226611201486633717649965547025203704833984375;-0.04411913978925187385105033399668172933161258697509765625;-0.80782568682606725740669162405538372695446014404296875;-0.6200953609438595304226282678428106009960174560546875;0.166911572703098476377903125467128120362758636474609375;-0.67251691842232352858133026529685594141483306884765625;-0.71180045685606330163608390648732893168926239013671875;0.1965578885687979393548374673628131859004497528076171875]
      mask Display: e = 0.06;c1 = [120 150 230]/255;c2 = ([120 150 230]+0)/383;c3 = ([120 150 230]+128)/383;patch([0 1 1 0],[0 0 1 1],c1);patch([0 1 1 1-e 1-e 0+e],[0 0 1 1-e 0+e 0+e],c2);patch([0 0 1 1-e 0+e 0+e],[0 1 1 1-e 1-e 0+e],c3);plot([0 1 1 0 0],[0 0 1 1 0]);disp('weights');
  "IW{5,4}(5,:)'" : Constant  Value=[0.98996669611439236380334705245331861078739166259765625;-0.68608390137380670381617164821363985538482666015625;0.522083386618934941481029454735107719898223876953125;0.82822397845458317622302502059028483927249908447265625;0.4391395410114122821454429868026636540889739990234375;-0.2127873190922124069235366050634183920919895172119140625;0.048569285738772817462294284496238105930387973785400390625;0.71502589165081620325992162179318256676197052001953125;-0.2995308731423136361371462044189684092998504638671875;0.2811720937549264665022974440944381058216094970703125;1.09360480022623551832339217071421444416046142578125;0.2684888737236927891416371494415216147899627685546875;-0.85098612588951760837829851880087517201900482177734375;-0.99906068019904747945503231676411814987659454345703125;-0.7962914572423465120465380095993168652057647705078125;-0.9950624259413773931015612106421031057834625244140625;-0.81846926967909627848030140739865601062774658203125;0.1439225314429584401398898307888885028660297393798828125;-0.1574681634601291790875876586142112500965595245361328125;0.79137319079697399093475951303844340145587921142578125]
      mask Display: e = 0.06;c1 = [120 150 230]/255;c2 = ([120 150 230]+0)/383;c3 = ([120 150 230]+128)/383;patch([0 1 1 0],[0 0 1 1],c1);patch([0 1 1 1-e 1-e 0+e],[0 0 1 1-e 0+e 0+e],c2);patch([0 0 1 1-e 0+e 0+e],[0 1 1 1-e 1-e 0+e],c3);plot([0 1 1 0 0],[0 0 1 1 0]);disp('weights');
  Mux : Mux  Inputs=5
      mask Display: e = 0.06;c1 = [120 150 230]/255;c2 = ([120 150 230]+0)/383;c3 = ([120 150 230]+128)/383;patch([0 1 1 0],[0 0 1 1],c1);patch([0 1 1 1-e 1-e 0+e],[0 0 1 1-e 0+e 0+e],c2);patch([0 0 1 1-e 0+e 0+e],[0 1 1 1-e 1-e 0+e],c3);plot([0 1 1 0 0],[0 0 1 1 0]);disp('Mux');
  dotprod{1..5} (5 alike) : neural/Weight Functions/dotprod
  "lz{5,4}" : Outport
      mask Display: e = 0.06;c1 = [120 230 180]/255;c2 = ([120 230 180]+0)/(256+128);c3 = ([120 230 180]+128)/(256+128);patch([0 1 1 0],[0 0 1 1],c1);patch([0 1 1 1-e 1-e 0+e],[0 0 1 1-e 0+e 0+e],c2);patch([0 0 1 1-e 0+e 0+e],[0 1 1 1-e 1-e 0+e],c3);plot([0 1 1 0 0],[0 0 1 1 0]);
  wires:
  Mux/1 -> "lz{5,4}"/1
  dotprod5/1 -> Mux/5
  "IW{5,4}(5,:)'"/1 -> dotprod5/1
  dotprod4/1 -> Mux/4
  "IW{5,4}(4,:)'"/1 -> dotprod4/1
  dotprod3/1 -> Mux/3
  "IW{5,4}(3,:)'"/1 -> dotprod3/1
  dotprod2/1 -> Mux/2
  "IW{5,4}(2,:)'"/1 -> dotprod2/1
  dotprod1/1 -> Mux/1
  "ad{5,4}"/1 -> dotprod5/2, dotprod4/2, dotprod3/2, dotprod2/2, dotprod1/2
  "IW{5,4}(1,:)'"/1 -> dotprod1/1

== system My_Model/Subsystem1/Custom Neural Network1/Layer 6/Delays 1 ==
  "p{6}" : Inport  PortDimensions=2
      mask Display: e = 0.06;c1 = [120 230 180]/255;c2 = ([120 230 180]+0)/(256+128);c3 = ([120 230 180]+128)/(256+128);patch([0 1 1 0],[0 0 1 1],c1);patch([0 1 1 1-e 1-e 0+e],[0 0 1 1-e 0+e 0+e],c2);patch([0 0 1 1-e 0+e 0+e],[0 1 1 1-e 1-e 0+e],c3);plot([0 1 1 0 0],[0 0 1 1 0]);
  mux : Mux  Inputs=1
      mask Display: e = 0.06;c1 = [120 150 230]/255;c2 = ([120 150 230]+0)/383;c3 = ([120 150 230]+128)/383;patch([0 1 1 0],[0 0 1 1],c1);patch([0 1 1 1-e 1-e 0+e],[0 0 1 1-e 0+e 0+e],c2);patch([0 0 1 1-e 0+e 0+e],[0 1 1 1-e 1-e 0+e],c3);plot([0 1 1 0 0],[0 0 1 1 0]);disp('Mux')
  "pd{6,1}" : Outport
      mask Display: e = 0.06;c1 = [120 230 180]/255;c2 = ([120 230 180]+0)/(256+128);c3 = ([120 230 180]+128)/(256+128);patch([0 1 1 0],[0 0 1 1],c1);patch([0 1 1 1-e 1-e 0+e],[0 0 1 1-e 0+e 0+e],c2);patch([0 0 1 1-e 0+e 0+e],[0 1 1 1-e 1-e 0+e],c3);plot([0 1 1 0 0],[0 0 1 1 0]);
  wires:
  mux/1 -> "pd{6,1}"/1
  "p{6}"/1 -> mux/1

== system My_Model/Subsystem1/Custom Neural Network1/Layer 6/Delays 2 ==
  "p{6}" : Inport  PortDimensions=5
      mask Display: e = 0.06;c1 = [120 230 180]/255;c2 = ([120 230 180]+0)/(256+128);c3 = ([120 230 180]+128)/(256+128);patch([0 1 1 0],[0 0 1 1],c1);patch([0 1 1 1-e 1-e 0+e],[0 0 1 1-e 0+e 0+e],c2);patch([0 0 1 1-e 0+e 0+e],[0 1 1 1-e 1-e 0+e],c3);plot([0 1 1 0 0],[0 0 1 1 0]);
  mux : Mux  Inputs=1
      mask Display: e = 0.06;c1 = [120 150 230]/255;c2 = ([120 150 230]+0)/383;c3 = ([120 150 230]+128)/383;patch([0 1 1 0],[0 0 1 1],c1);patch([0 1 1 1-e 1-e 0+e],[0 0 1 1-e 0+e 0+e],c2);patch([0 0 1 1-e 0+e 0+e],[0 1 1 1-e 1-e 0+e],c3);plot([0 1 1 0 0],[0 0 1 1 0]);disp('Mux')
  "pd{6,1}" : Outport
      mask Display: e = 0.06;c1 = [120 230 180]/255;c2 = ([120 230 180]+0)/(256+128);c3 = ([120 230 180]+128)/(256+128);patch([0 1 1 0],[0 0 1 1],c1);patch([0 1 1 1-e 1-e 0+e],[0 0 1 1-e 0+e 0+e],c2);patch([0 0 1 1-e 0+e 0+e],[0 1 1 1-e 1-e 0+e],c3);plot([0 1 1 0 0],[0 0 1 1 0]);
  wires:
  mux/1 -> "pd{6,1}"/1
  "p{6}"/1 -> mux/1

== system My_Model/Subsystem1/Custom Neural Network1/Layer 6/Delays 3 ==
  "p{6}" : Inport  PortDimensions=20
      mask Display: e = 0.06;c1 = [120 230 180]/255;c2 = ([120 230 180]+0)/(256+128);c3 = ([120 230 180]+128)/(256+128);patch([0 1 1 0],[0 0 1 1],c1);patch([0 1 1 1-e 1-e 0+e],[0 0 1 1-e 0+e 0+e],c2);patch([0 0 1 1-e 0+e 0+e],[0 1 1 1-e 1-e 0+e],c3);plot([0 1 1 0 0],[0 0 1 1 0]);
  mux : Mux  Inputs=1
      mask Display: e = 0.06;c1 = [120 150 230]/255;c2 = ([120 150 230]+0)/383;c3 = ([120 150 230]+128)/383;patch([0 1 1 0],[0 0 1 1],c1);patch([0 1 1 1-e 1-e 0+e],[0 0 1 1-e 0+e 0+e],c2);patch([0 0 1 1-e 0+e 0+e],[0 1 1 1-e 1-e 0+e],c3);plot([0 1 1 0 0],[0 0 1 1 0]);disp('Mux')
  "pd{6,2}" : Outport
      mask Display: e = 0.06;c1 = [120 230 180]/255;c2 = ([120 230 180]+0)/(256+128);c3 = ([120 230 180]+128)/(256+128);patch([0 1 1 0],[0 0 1 1],c1);patch([0 1 1 1-e 1-e 0+e],[0 0 1 1-e 0+e 0+e],c2);patch([0 0 1 1-e 0+e 0+e],[0 1 1 1-e 1-e 0+e],c3);plot([0 1 1 0 0],[0 0 1 1 0]);
  wires:
  mux/1 -> "pd{6,2}"/1
  "p{6}"/1 -> mux/1

== system My_Model/Subsystem1/Custom Neural Network1/Layer 6/Delays 4 ==
  "p{6}" : Inport  PortDimensions=30
      mask Display: e = 0.06;c1 = [120 230 180]/255;c2 = ([120 230 180]+0)/(256+128);c3 = ([120 230 180]+128)/(256+128);patch([0 1 1 0],[0 0 1 1],c1);patch([0 1 1 1-e 1-e 0+e],[0 0 1 1-e 0+e 0+e],c2);patch([0 0 1 1-e 0+e 0+e],[0 1 1 1-e 1-e 0+e],c3);plot([0 1 1 0 0],[0 0 1 1 0]);
  mux : Mux  Inputs=1
      mask Display: e = 0.06;c1 = [120 150 230]/255;c2 = ([120 150 230]+0)/383;c3 = ([120 150 230]+128)/383;patch([0 1 1 0],[0 0 1 1],c1);patch([0 1 1 1-e 1-e 0+e],[0 0 1 1-e 0+e 0+e],c2);patch([0 0 1 1-e 0+e 0+e],[0 1 1 1-e 1-e 0+e],c3);plot([0 1 1 0 0],[0 0 1 1 0]);disp('Mux')
  "pd{6,3}" : Outport
      mask Display: e = 0.06;c1 = [120 230 180]/255;c2 = ([120 230 180]+0)/(256+128);c3 = ([120 230 180]+128)/(256+128);patch([0 1 1 0],[0 0 1 1],c1);patch([0 1 1 1-e 1-e 0+e],[0 0 1 1-e 0+e 0+e],c2);patch([0 0 1 1-e 0+e 0+e],[0 1 1 1-e 1-e 0+e],c3);plot([0 1 1 0 0],[0 0 1 1 0]);
  wires:
  mux/1 -> "pd{6,3}"/1
  "p{6}"/1 -> mux/1

== system My_Model/Subsystem1/Custom Neural Network1/Layer 6/Delays 5 ==
  "p{6}" : Inport  PortDimensions=20
      mask Display: e = 0.06;c1 = [120 230 180]/255;c2 = ([120 230 180]+0)/(256+128);c3 = ([120 230 180]+128)/(256+128);patch([0 1 1 0],[0 0 1 1],c1);patch([0 1 1 1-e 1-e 0+e],[0 0 1 1-e 0+e 0+e],c2);patch([0 0 1 1-e 0+e 0+e],[0 1 1 1-e 1-e 0+e],c3);plot([0 1 1 0 0],[0 0 1 1 0]);
  mux : Mux  Inputs=1
      mask Display: e = 0.06;c1 = [120 150 230]/255;c2 = ([120 150 230]+0)/383;c3 = ([120 150 230]+128)/383;patch([0 1 1 0],[0 0 1 1],c1);patch([0 1 1 1-e 1-e 0+e],[0 0 1 1-e 0+e 0+e],c2);patch([0 0 1 1-e 0+e 0+e],[0 1 1 1-e 1-e 0+e],c3);plot([0 1 1 0 0],[0 0 1 1 0]);disp('Mux')
  "pd{6,4}" : Outport
      mask Display: e = 0.06;c1 = [120 230 180]/255;c2 = ([120 230 180]+0)/(256+128);c3 = ([120 230 180]+128)/(256+128);patch([0 1 1 0],[0 0 1 1],c1);patch([0 1 1 1-e 1-e 0+e],[0 0 1 1-e 0+e 0+e],c2);patch([0 0 1 1-e 0+e 0+e],[0 1 1 1-e 1-e 0+e],c3);plot([0 1 1 0 0],[0 0 1 1 0]);
  wires:
  mux/1 -> "pd{6,4}"/1
  "p{6}"/1 -> mux/1

== system My_Model/Subsystem1/Custom Neural Network1/Layer 6/Delays 6 ==
  "p{6}" : Inport  PortDimensions=5
      mask Display: e = 0.06;c1 = [120 230 180]/255;c2 = ([120 230 180]+0)/(256+128);c3 = ([120 230 180]+128)/(256+128);patch([0 1 1 0],[0 0 1 1],c1);patch([0 1 1 1-e 1-e 0+e],[0 0 1 1-e 0+e 0+e],c2);patch([0 0 1 1-e 0+e 0+e],[0 1 1 1-e 1-e 0+e],c3);plot([0 1 1 0 0],[0 0 1 1 0]);
  mux : Mux  Inputs=1
      mask Display: e = 0.06;c1 = [120 150 230]/255;c2 = ([120 150 230]+0)/383;c3 = ([120 150 230]+128)/383;patch([0 1 1 0],[0 0 1 1],c1);patch([0 1 1 1-e 1-e 0+e],[0 0 1 1-e 0+e 0+e],c2);patch([0 0 1 1-e 0+e 0+e],[0 1 1 1-e 1-e 0+e],c3);plot([0 1 1 0 0],[0 0 1 1 0]);disp('Mux')
  "pd{6,5}" : Outport
      mask Display: e = 0.06;c1 = [120 230 180]/255;c2 = ([120 230 180]+0)/(256+128);c3 = ([120 230 180]+128)/(256+128);patch([0 1 1 0],[0 0 1 1],c1);patch([0 1 1 1-e 1-e 0+e],[0 0 1 1-e 0+e 0+e],c2);patch([0 0 1 1-e 0+e 0+e],[0 1 1 1-e 1-e 0+e],c3);plot([0 1 1 0 0],[0 0 1 1 0]);
  wires:
  mux/1 -> "pd{6,5}"/1
  "p{6}"/1 -> mux/1

== system My_Model/Subsystem1/Custom Neural Network1/Layer 6/IW{6,1} ==
  "pd{6,1}" : Inport  PortDimensions=2
      mask Display: e = 0.06;c1 = [120 230 180]/255;c2 = ([120 230 180]+0)/(256+128);c3 = ([120 230 180]+128)/(256+128);patch([0 1 1 0],[0 0 1 1],c1);patch([0 1 1 1-e 1-e 0+e],[0 0 1 1-e 0+e 0+e],c2);patch([0 0 1 1-e 0+e 0+e],[0 1 1 1-e 1-e 0+e],c3);plot([0 1 1 0 0],[0 0 1 1 0]);
  "IW{6,1}(1,:)'" : Constant  Value=[0.055896275110062960955747968228024546988308429718017578125;-0.434678222920332368861551231020712293684482574462890625]
      mask Display: e = 0.06;c1 = [120 150 230]/255;c2 = ([120 150 230]+0)/383;c3 = ([120 150 230]+128)/383;patch([0 1 1 0],[0 0 1 1],c1);patch([0 1 1 1-e 1-e 0+e],[0 0 1 1-e 0+e 0+e],c2);patch([0 0 1 1-e 0+e 0+e],[0 1 1 1-e 1-e 0+e],c3);plot([0 1 1 0 0],[0 0 1 1 0]);disp('Weights');
  Mux : Mux  Inputs=1
      mask Display: e = 0.06;c1 = [120 150 230]/255;c2 = ([120 150 230]+0)/383;c3 = ([120 150 230]+128)/383;patch([0 1 1 0],[0 0 1 1],c1);patch([0 1 1 1-e 1-e 0+e],[0 0 1 1-e 0+e 0+e],c2);patch([0 0 1 1-e 0+e 0+e],[0 1 1 1-e 1-e 0+e],c3);plot([0 1 1 0 0],[0 0 1 1 0]);disp('Mux');
  dotprod1 : neural/Weight Functions/dotprod
  "iz{6,1}" : Outport
      mask Display: e = 0.06;c1 = [120 230 180]/255;c2 = ([120 230 180]+0)/(256+128);c3 = ([120 230 180]+128)/(256+128);patch([0 1 1 0],[0 0 1 1],c1);patch([0 1 1 1-e 1-e 0+e],[0 0 1 1-e 0+e 0+e],c2);patch([0 0 1 1-e 0+e 0+e],[0 1 1 1-e 1-e 0+e],c3);plot([0 1 1 0 0],[0 0 1 1 0]);
  wires:
  Mux/1 -> "iz{6,1}"/1
  dotprod1/1 -> Mux/1
  "pd{6,1}"/1 -> dotprod1/2
  "IW{6,1}(1,:)'"/1 -> dotprod1/1

== system My_Model/Subsystem1/Custom Neural Network1/Layer 6/LW{6,1} ==
  "ad{6,1}" : Inport  PortDimensions=5
      mask Display: e = 0.06;c1 = [120 230 180]/255;c2 = ([120 230 180]+0)/(256+128);c3 = ([120 230 180]+128)/(256+128);patch([0 1 1 0],[0 0 1 1],c1);patch([0 1 1 1-e 1-e 0+e],[0 0 1 1-e 0+e 0+e],c2);patch([0 0 1 1-e 0+e 0+e],[0 1 1 1-e 1-e 0+e],c3);plot([0 1 1 0 0],[0 0 1 1 0]);
  "IW{6,1}(1,:)'" : Constant  Value=[0.06866122477737866824920587305314256809651851654052734375;0.387105716830645596449045342524186708033084869384765625;-0.6764176634318561642800204936065711081027984619140625;0.0381756012822151713503870951171847991645336151123046875;0.1618969824994793416106375616436707787215709686279296875]
      mask Display: e = 0.06;c1 = [120 150 230]/255;c2 = ([120 150 230]+0)/383;c3 = ([120 150 230]+128)/383;patch([0 1 1 0],[0 0 1 1],c1);patch([0 1 1 1-e 1-e 0+e],[0 0 1 1-e 0+e 0+e],c2);patch([0 0 1 1-e 0+e 0+e],[0 1 1 1-e 1-e 0+e],c3);plot([0 1 1 0 0],[0 0 1 1 0]);disp('weights');
  Mux : Mux  Inputs=1
      mask Display: e = 0.06;c1 = [120 150 230]/255;c2 = ([120 150 230]+0)/383;c3 = ([120 150 230]+128)/383;patch([0 1 1 0],[0 0 1 1],c1);patch([0 1 1 1-e 1-e 0+e],[0 0 1 1-e 0+e 0+e],c2);patch([0 0 1 1-e 0+e 0+e],[0 1 1 1-e 1-e 0+e],c3);plot([0 1 1 0 0],[0 0 1 1 0]);disp('Mux');
  dotprod1 : neural/Weight Functions/dotprod
  "lz{6,1}" : Outport
      mask Display: e = 0.06;c1 = [120 230 180]/255;c2 = ([120 230 180]+0)/(256+128);c3 = ([120 230 180]+128)/(256+128);patch([0 1 1 0],[0 0 1 1],c1);patch([0 1 1 1-e 1-e 0+e],[0 0 1 1-e 0+e 0+e],c2);patch([0 0 1 1-e 0+e 0+e],[0 1 1 1-e 1-e 0+e],c3);plot([0 1 1 0 0],[0 0 1 1 0]);
  wires:
  Mux/1 -> "lz{6,1}"/1
  dotprod1/1 -> Mux/1
  "ad{6,1}"/1 -> dotprod1/2
  "IW{6,1}(1,:)'"/1 -> dotprod1/1

== system My_Model/Subsystem1/Custom Neural Network1/Layer 6/LW{6,2} ==
  "ad{6,2}" : Inport  PortDimensions=20
      mask Display: e = 0.06;c1 = [120 230 180]/255;c2 = ([120 230 180]+0)/(256+128);c3 = ([120 230 180]+128)/(256+128);patch([0 1 1 0],[0 0 1 1],c1);patch([0 1 1 1-e 1-e 0+e],[0 0 1 1-e 0+e 0+e],c2);patch([0 0 1 1-e 0+e 0+e],[0 1 1 1-e 1-e 0+e],c3);plot([0 1 1 0 0],[0 0 1 1 0]);
  "IW{6,2}(1,:)'" : Constant  Value=[0.43108010730528512066683788361842744052410125732421875;-0.235408006018248239232804053244763053953647613525390625;0.5237222204917484358333013005903922021389007568359375;-0.60541251309444577000107301500975154340267181396484375;0.470567080829956407850289679117850027978420257568359375;0.2707873223901609005537238772376440465450286865234375;0.06424567495048620624498170172955724410712718963623046875;0.682682123190482936792022883309982717037200927734375;-0.8503104178633387189023551400168798863887786865234375;0.21341363749515840364523455718881450593471527099609375;0.65503603031855861527077422579168342053890228271484375;0.448304336271322101392655667950748465955257415771484375;0.318090895673833473633607127339928410947322845458984375;0.55948095721561441617808441151282750070095062255859375;0.42255206382583609947545255636214278638362884521484375;-0.262936674498417011225370742977247573435306549072265625;0.11132424169928763213466282877561752684414386749267578125;0.90894434072684682224263497118954546749591827392578125;-0.6458440127441200662161691070650704205036163330078125;0.376115433379758890009014749011839739978313446044921875]
      mask Display: e = 0.06;c1 = [120 150 230]/255;c2 = ([120 150 230]+0)/383;c3 = ([120 150 230]+128)/383;patch([0 1 1 0],[0 0 1 1],c1);patch([0 1 1 1-e 1-e 0+e],[0 0 1 1-e 0+e 0+e],c2);patch([0 0 1 1-e 0+e 0+e],[0 1 1 1-e 1-e 0+e],c3);plot([0 1 1 0 0],[0 0 1 1 0]);disp('weights');
  Mux : Mux  Inputs=1
      mask Display: e = 0.06;c1 = [120 150 230]/255;c2 = ([120 150 230]+0)/383;c3 = ([120 150 230]+128)/383;patch([0 1 1 0],[0 0 1 1],c1);patch([0 1 1 1-e 1-e 0+e],[0 0 1 1-e 0+e 0+e],c2);patch([0 0 1 1-e 0+e 0+e],[0 1 1 1-e 1-e 0+e],c3);plot([0 1 1 0 0],[0 0 1 1 0]);disp('Mux');
  dotprod1 : neural/Weight Functions/dotprod
  "lz{6,2}" : Outport
      mask Display: e = 0.06;c1 = [120 230 180]/255;c2 = ([120 230 180]+0)/(256+128);c3 = ([120 230 180]+128)/(256+128);patch([0 1 1 0],[0 0 1 1],c1);patch([0 1 1 1-e 1-e 0+e],[0 0 1 1-e 0+e 0+e],c2);patch([0 0 1 1-e 0+e 0+e],[0 1 1 1-e 1-e 0+e],c3);plot([0 1 1 0 0],[0 0 1 1 0]);
  wires:
  Mux/1 -> "lz{6,2}"/1
  dotprod1/1 -> Mux/1
  "ad{6,2}"/1 -> dotprod1/2
  "IW{6,2}(1,:)'"/1 -> dotprod1/1
